simulink model "OUR_BD_FUELCELL"  (R2022b)
settings: Solver=ode1  StartTime=0.0  StopTime=max(cyc_mph(:,1))  FixedStep=1  MaxStep=1  RelTol=1e-3  AbsTol=1e-3
values from neighbouring files (symbols this model uses):
  eta_DC_DC = 1    [main.m]
  fc_pwr_scale = 0.6    [fuelcell_patch.m]
  Ts = 1    [main.m]
undefined symbols (not defined in the file or in its folder): air_cp, amb_tmp, cs_charge_deplete_bool, cs_charge_pwr, cs_fc_init_state, cs_fc_on, cs_hi_soc, cs_lo_soc, cs_max_pwr, cs_max_pwr_fall_rate, cs_max_pwr_rise_rate, cs_min_off_time, cs_min_pwr, ess_on, ex_calc, ex_gas_cp, fc_acc_mass, fc_base_mass, fc_c2i_th_cond, fc_c_init_tmp, fc_cl2h_eff, fc_co_map, fc_co_map_c2h, fc_cold, fc_cold_tmp, fc_cp, fc_eff_scale, fc_emis, fc_emisv, fc_exflow_map, fc_ext_sarea, fc_extmp_map, fc_fuel_den, fc_fuel_lhv, fc_fuel_map, fc_fuel_map_c2h, fc_fuelcell_warmup_bool, fc_h2x_th_cond, fc_h_air_flow, fc_h_cp, fc_h_init_tmp, fc_hc_map, fc_hc_map_c2h, fc_hood_emisv, fc_hood_sarea, fc_i2x_th_cond, fc_i_init_tmp, fc_nox_map, fc_nox_map_c2h, fc_o2_map, fc_on, fc_pm_map, fc_pm_map_c2h, fc_pwr_map, fc_tstat, fc_x_init_tmp, pow, veh_glider_mass
libraries: lib_wheel x2, lib_help x2, lib_transmission x2, lib_outputs x1, lib_controls x1, lib_interactive x1, lib_drive_cycle x1, lib_accessory x1, lib_energy_storage x1, lib_exhaust x1, mpclib x1, lib_electric_machine x1
(part 2 of 2)

== system OUR_BD_FUELCELL/fuel converter <fc> net model/fuel use and EO emis Fuel Cell/fc temp correct ==
  Coolant T (C) : Inport
  HOT fuel use (g/s) : Inport  Port=2
  HOT emis (g/s) : Inport  Port=3
  P (W) : Inport  Port=4
  Enable : EnablePort  StatesWhenEnabling=reset
  =1: use map based =0: use constant equation based : Constant  Value=fc_cold
  Switch : Switch  Threshold=eps
  Switch1 : Switch  Threshold=eps
  fc temp correct Constant Correction Factors (Equation Based) : Subsystem  TreatAsAtomicUnit=on
  fc temp correct Variable Correction Factors (Map Based) : Subsystem  TreatAsAtomicUnit=on
  fc_cold=0 : Logic  Operator=NOT
  fuel use (g/s) : Outport  OutputWhenDisabled=reset  InitialOutput=0
  EO emis (g/s) : Outport  Port=2  OutputWhenDisabled=reset  InitialOutput=0
  wires:
  Switch1/1 -> EO emis (g/s)/1
  Switch/1 -> fuel use (g/s)/1
  fc temp correct Variable Correction Factors (Map Based)/2(EO emis (g/s)) -> Switch1/3
  fc temp correct Constant Correction Factors (Equation Based)/2(EO emis (g/s)) -> Switch1/1
  fc temp correct Variable Correction Factors (Map Based)/1(fuel use (g/s)) -> Switch/3
  fc_cold=0/1 -> Switch1/2, Switch/2, fc temp correct Constant Correction Factors (Equation Based)/Enable
  fc temp correct Constant Correction Factors (Equation Based)/1(fuel use (g/s)) -> Switch/1
  HOT emis (g/s)/1 -> fc temp correct Variable Correction Factors (Map Based)/3(HOT emis (g/s)), fc temp correct Constant Correction Factors (Equation Based)/3(HOT emis (g/s))
  HOT fuel use (g/s)/1 -> fc temp correct Variable Correction Factors (Map Based)/2(HOT fuel use (g/s)), fc temp correct Constant Correction Factors (Equation Based)/2(HOT fuel use (g/s))
  Coolant T (C)/1 -> fc temp correct Variable Correction Factors (Map Based)/1(Coolant T (C)), fc temp correct Constant Correction Factors (Equation Based)/1(Coolant T (C))
  =1: use map based =0: use constant equation based/1 -> fc temp correct Variable Correction Factors (Map Based)/Enable, fc_cold=0/1
  P (W)/1 -> fc temp correct Variable Correction Factors (Map Based)/4(P (W))

== system OUR_BD_FUELCELL/fuel cell control strategy <cs>/FC on/no-lag Reset Integrator/dt ==
  Clock : Clock
  Memory1 : Memory  InitialCondition=-1
  Sum1 : Sum  Inputs=+-  InputSameDT=on  SaturateOnIntegerOverflow=on  OutDataTypeStr=Inherit: Same as first input
  out_1 : Outport  InitialOutput=0
  wires:
  Sum1/1 -> out_1/1
  Memory1/1 -> Sum1/2
  Clock/1 -> Memory1/1, Sum1/1

== system OUR_BD_FUELCELL/fuel cell control strategy <cs>/FC on1/no-lag Reset Integrator/dt ==
  Clock : Clock
  Memory1 : Memory  InitialCondition=-1
  Sum1 : Sum  Inputs=+-  InputSameDT=on  SaturateOnIntegerOverflow=on  OutDataTypeStr=Inherit: Same as first input
  out_1 : Outport  InitialOutput=0
  wires:
  Sum1/1 -> out_1/1
  Memory1/1 -> Sum1/2
  Clock/1 -> Memory1/1, Sum1/1

== system OUR_BD_FUELCELL/fuel converter <fc> net model/fuel cell system <fc>/pwr vs. eff fuel cell model/enforce limits ==
  In1 : Inport
  Gain : Gain  Gain=eta_DC_DC
  Saturation : Saturate  UpperLimit=max(fc_pwr_map)*fc_pwr_scale  LowerLimit=0
  Out1 : Outport  InitialOutput=0
  wires:
  In1/1 -> Saturation/1
  Saturation/1 -> Gain/1
  Gain/1 -> Out1/1

== system OUR_BD_FUELCELL/fuel converter <fc> net model/fuel use and EO emis Fuel Cell/HOT engine maps /Block NOTES ==
  note: This block determines the fully hot fuel use, engine-out emissions output rates, exhaust gas mass flow rate,
      | and engine-out exhaust gas temperature as a function of engine output torque and speed.
      | The engine maps (except for exhaust gas temperature) can be scaled using variables fc_spd_scale and
      |  fc_trq_scale; it is recommended that scaling values outside the range of 0.85 to 1.15 be used CAREFULLY.

== system OUR_BD_FUELCELL/fuel converter <fc> net model/fuel use and EO emis Fuel Cell/fc temp/Block NOTES ==
  note: This block models the thermal behavior internal combustion engine (ICE).
      | Emphasis is on the coolant since this temperature is used to correct engine
      | fuel use.

== system OUR_BD_FUELCELL/fuel converter <fc> net model/fuel use and EO emis Fuel Cell/fc temp/fc coolant ==
  Tcl : Inport
  "Qfc_i " : Inport  Port=2
  Enable : EnablePort  StatesWhenEnabling=reset
  Constant : Constant  Value=fc_tstat
  Product1 : Product  InputSameDT=on  RndMeth=Zero  SaturateOnIntegerOverflow=on  OutDataTypeStr=Inherit: Same as first input
  Qhtr : Fcn  Expr=fc_cl2h_eff*fc_h_air_flow*air_cp*(u - amb_tmp)
  Qi : Sum  Inputs=-+  InputSameDT=on  SaturateOnIntegerOverflow=on  OutDataTypeStr=Inherit: Same as first input
  Relational Operator : RelationalOperator  Operator=<=
  Qfc_rad : Outport  OutputWhenDisabled=reset  InitialOutput=0
  Qfc_htr : Outport  Port=2  OutputWhenDisabled=reset  InitialOutput=0
  wires:
  Qi/1 -> Product1/2
  Qhtr/1 -> Qfc_htr/1, Qi/1
  "Qfc_i "/1 -> Qi/2
  Product1/1 -> Qfc_rad/1
  Constant/1 -> Relational Operator/1
  Relational Operator/1 -> Product1/1
  Tcl/1 -> Relational Operator/2, Qhtr/1

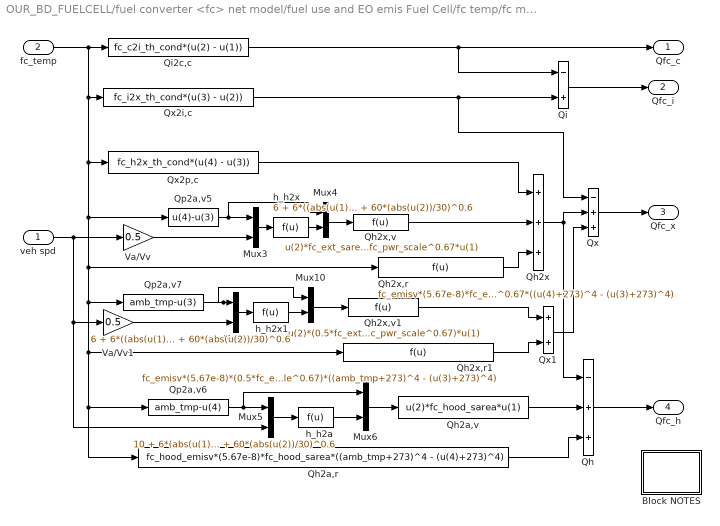
== system OUR_BD_FUELCELL/fuel converter <fc> net model/fuel use and EO emis Fuel Cell/fc temp/fc mass heat flow ==
  veh spd : Inport
  fc_temp : Inport  Port=2
  Block NOTES : Subsystem
      mask Display: disp('Block\nNOTES')
  Mux{3..6,9..10} (6 alike) : Mux  Inputs=2
  Qh : Sum  Inputs=-++  InputSameDT=on  SaturateOnIntegerOverflow=on  OutDataTypeStr=Inherit: Same as first input
  Qh2a,r : Fcn  Expr=fc_hood_emisv*(5.67e-8)*fc_hood_sarea*((amb_tmp+273)^4 - (u(4)+273)^4)
  Qh2a,v : Fcn  Expr=u(2)*fc_hood_sarea*u(1)
  Qh2x : Sum  Inputs=+++  InputSameDT=on  SaturateOnIntegerOverflow=on  OutDataTypeStr=Inherit: Same as first input
  Qh2x,r : Fcn  Expr=fc_emisv*(5.67e-8)*fc_ext_sarea*fc_pwr_scale^0.67*((u(4)+273)^4 - (u(3)+273)^4)
  Qh2x,r1 : Fcn  Expr=fc_emisv*(5.67e-8)*(0.5*fc_ext_sarea*fc_pwr_scale^0.67)*((amb_tmp+273)^4 - (u(3)+273)^4)
  Qh2x,v : Fcn  Expr=u(2)*fc_ext_sarea*fc_pwr_scale^0.67*u(1)
  Qh2x,v1 : Fcn  Expr=u(2)*(0.5*fc_ext_sarea*fc_pwr_scale^0.67)*u(1)
  Qi : Sum  Inputs=-+  InputSameDT=on  SaturateOnIntegerOverflow=on  OutDataTypeStr=Inherit: Same as first input
  Qi2c,c : Fcn  Expr=fc_c2i_th_cond*(u(2) - u(1))
  Qp2a,v5 : Fcn  Expr=u(4)-u(3)
  Qp2a,v6 : Fcn  Expr=amb_tmp-u(4)
  Qp2a,v7 : Fcn  Expr=amb_tmp-u(3)
  Qx : Sum  Inputs=-++  InputSameDT=on  SaturateOnIntegerOverflow=on  OutDataTypeStr=Inherit: Same as first input
  Qx1 : Sum  InputSameDT=on  SaturateOnIntegerOverflow=on  OutDataTypeStr=Inherit: Same as first input
  Qx2i,c : Fcn  Expr=fc_i2x_th_cond*(u(3) - u(2))
  Qx2p,c : Fcn  Expr=fc_h2x_th_cond*(u(4) - u(3))
  Va/Vv : Gain  Gain=0.5  SaturateOnIntegerOverflow=on  OutDataTypeStr=Inherit: Same as input  ParamDataTypeStr=Inherit: Same as input
  Va/Vv1 : Gain  Gain=0.5  SaturateOnIntegerOverflow=on  OutDataTypeStr=Inherit: Same as input  ParamDataTypeStr=Inherit: Same as input
  h_h2a : Fcn  Expr=10 + 6*(abs(u(1))/1000)^0.3 + 60*(abs(u(2))/30)^0.6
  h_h2x : Fcn  Expr=6 + 6*((abs(u(1))/1000))^0.3 + 60*(abs(u(2))/30)^0.6
  h_h2x1 : Fcn  Expr=6 + 6*((abs(u(1))/1000))^0.3 + 60*(abs(u(2))/30)^0.6
  Qfc_c : Outport
  Qfc_i : Outport  Port=2
  Qfc_x : Outport  Port=3
  Qfc_h : Outport  Port=4
  wires:
  Qh2x,r/1 -> Qh2x/3
  Qh2a,v/1 -> Qh/2
  Qh2a,r/1 -> Qh/3
  Qh2x,v1/1 -> Qx1/1
  Qh2x,r1/1 -> Qx1/2
  Qx2p,c/1 -> Qh2x/1
  Qh2x,v/1 -> Qh2x/2
  Qx1/1 -> Qx/3
  h_h2a/1 -> Mux6/2
  Qp2a,v6/1 -> Mux6/1, Mux5/1
  Mux5/1 -> h_h2a/1
  Mux6/1 -> Qh2a,v/1
  Qh/1 -> Qfc_h/1
  Qh2x/1 -> Qh/1, Qx/2
  Qx/1 -> Qfc_x/1
  Qi/1 -> Qfc_i/1
  Qx2i,c/1 -> Qx/1, Qi/2
  fc_temp/1 -> Qi2c,c/1, Qx2i,c/1, Qp2a,v5/1, Qh2x,r1/1, Qh2a,r/1, Qp2a,v6/1, Qp2a,v7/1, Qh2x,r/1, Qx2p,c/1
  Qi2c,c/1 -> Qi/1, Qfc_c/1
  Va/Vv/1 -> Mux3/2
  veh spd/1 -> Va/Vv1/1, Mux5/2, Va/Vv/1
  h_h2x/1 -> Mux4/2
  Qp2a,v5/1 -> Mux4/1, Mux3/1
  Mux3/1 -> h_h2x/1
  Mux4/1 -> Qh2x,v/1
  Va/Vv1/1 -> Mux9/2
  h_h2x1/1 -> Mux10/2
  Qp2a,v7/1 -> Mux10/1, Mux9/1
  Mux9/1 -> h_h2x1/1
  Mux10/1 -> Qh2x,v1/1

== system OUR_BD_FUELCELL/fuel converter <fc> net model/fuel use and EO emis Fuel Cell/fc temp/old fc coolant temp. (C) ==
  fc on? : Inport
  veh spd : Inport  Port=2
  Block NOTES : Subsystem
      mask Display: disp('Block\nNOTES')
  Mux : Mux
  TEC : Integrator  InitialCondition=fc_i_init_tmp
  compute engine dT/dt : Fcn  Expr=1.1*u[1]*(-u[2]/218)*(95-u[4])+(1-u[1])*u[3]*(u[4]-amb_tmp)
  gamma (takes v as input) : Fcn  Expr=(-8.22e-5*u+8.09e-6*4-1.45e-4)*.45
  log(1-40/75) : Constant  Value=-0.7621
  fc coolant temp (C) : Outport  InitialOutput=0
  wires:
  TEC/1 -> Mux/4, fc coolant temp (C)/1
  veh spd/1 -> gamma (takes v as input)/1
  fc on?/1 -> Mux/1
  Mux/1 -> compute engine dT/dt/1
  log(1-40/75)/1 -> Mux/2
  gamma (takes v as input)/1 -> Mux/3
  compute engine dT/dt/1 -> TEC/1

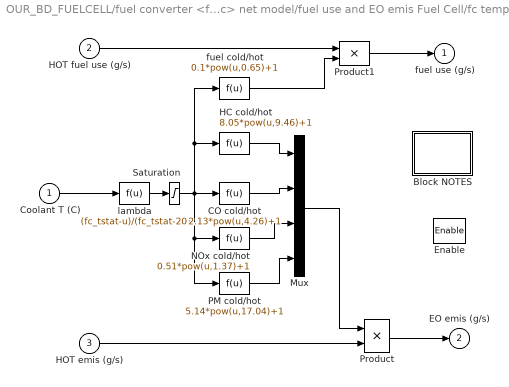
== system OUR_BD_FUELCELL/fuel converter <fc> net model/fuel use and EO emis Fuel Cell/fc temp correct/fc temp correct Constant Correction Factors (Equation Based) ==
  Coolant T (C) : Inport
  HOT fuel use (g/s) : Inport  Port=2
  HOT emis (g/s) : Inport  Port=3
  Enable : EnablePort  StatesWhenEnabling=reset
  Block NOTES : Subsystem
      mask Display: disp('Block\nNOTES')
  CO cold/hot : Fcn  Expr=2.13*pow(u,4.26)+1
  HC cold/hot : Fcn  Expr=8.05*pow(u,9.46)+1
  Mux : Mux
  NOx cold/hot : Fcn  Expr=0.51*pow(u,1.37)+1
  PM cold/hot : Fcn  Expr=5.14*pow(u,17.04)+1
  Product : Product  InputSameDT=on  RndMeth=Zero  SaturateOnIntegerOverflow=on  OutDataTypeStr=Inherit: Same as first input
  Product1 : Product  InputSameDT=on  RndMeth=Zero  SaturateOnIntegerOverflow=on  OutDataTypeStr=Inherit: Same as first input
  Saturation : Saturate  UpperLimit=1  LowerLimit=0
  fuel cold/hot : Fcn  Expr=0.1*pow(u,0.65)+1
  lambda : Fcn  Expr=(fc_tstat-u)/(fc_tstat-20)
  fuel use (g/s) : Outport  OutputWhenDisabled=reset  InitialOutput=0
  EO emis (g/s) : Outport  Port=2  OutputWhenDisabled=reset  InitialOutput=0
  wires:
  PM cold/hot/1 -> Mux/4
  NOx cold/hot/1 -> Mux/3
  HC cold/hot/1 -> Mux/1
  Saturation/1 -> CO cold/hot/1, HC cold/hot/1, fuel cold/hot/1, NOx cold/hot/1, PM cold/hot/1
  lambda/1 -> Saturation/1
  Mux/1 -> Product/1
  fuel cold/hot/1 -> Product1/2
  Product/1 -> EO emis (g/s)/1
  CO cold/hot/1 -> Mux/2
  Product1/1 -> fuel use (g/s)/1
  HOT fuel use (g/s)/1 -> Product1/1
  Coolant T (C)/1 -> lambda/1
  HOT emis (g/s)/1 -> Product/2

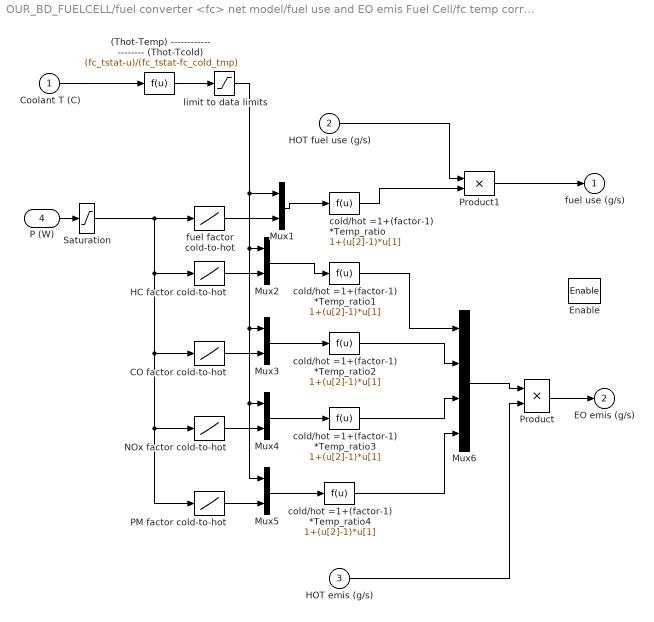
== system OUR_BD_FUELCELL/fuel converter <fc> net model/fuel use and EO emis Fuel Cell/fc temp correct/fc temp correct Variable Correction Factors (Map Based) ==
  Coolant T (C) : Inport
  HOT fuel use (g/s) : Inport  Port=2
  HOT emis (g/s) : Inport  Port=3
  P (W) : Inport  Port=4
  Enable : EnablePort  StatesWhenEnabling=reset
  (Thot-Temp) -------------------- (Thot-Tcold) : Fcn  Expr=(fc_tstat-u)/(fc_tstat-fc_cold_tmp)
  CO factor cold-to-hot : Lookup  InputValues=fc_pwr_map*fc_pwr_scale  Table=fc_co_map_c2h
  HC factor cold-to-hot : Lookup  InputValues=fc_pwr_map*fc_pwr_scale  Table=fc_hc_map_c2h
  Mux{1..5} (5 alike) : Mux  Inputs=2
  Mux6 : Mux
  NOx factor cold-to-hot : Lookup  InputValues=fc_pwr_map*fc_pwr_scale  Table=fc_nox_map_c2h
  PM factor cold-to-hot : Lookup  InputValues=fc_pwr_map*fc_pwr_scale  Table=fc_pm_map_c2h
  Product : Product  InputSameDT=on  RndMeth=Zero  SaturateOnIntegerOverflow=on  OutDataTypeStr=Inherit: Same as first input
  Product1 : Product  InputSameDT=on  RndMeth=Zero  SaturateOnIntegerOverflow=on  OutDataTypeStr=Inherit: Same as first input
  Saturation : Saturate  UpperLimit=max(fc_pwr_map*fc_pwr_scale)  LowerLimit=0
  cold/hot =1+(factor-1) *Temp_ratio{,1..4} (5 alike) : Fcn  Expr=1+(u[2]-1)*u[1]
  fuel factor cold-to-hot : Lookup  InputValues=fc_pwr_map*fc_pwr_scale  Table=fc_fuel_map_c2h
  limit to data limits : Saturate  UpperLimit=1  LowerLimit=0
  fuel use (g/s) : Outport  OutputWhenDisabled=reset  InitialOutput=0
  EO emis (g/s) : Outport  Port=2  OutputWhenDisabled=reset  InitialOutput=0
  wires:
  Mux6/1 -> Product/1
  HOT emis (g/s)/1 -> Product/2
  Product/1 -> EO emis (g/s)/1
  Product1/1 -> fuel use (g/s)/1
  Mux5/1 -> cold/hot =1+(factor-1) *Temp_ratio4/1
  Mux4/1 -> cold/hot =1+(factor-1) *Temp_ratio3/1
  Mux3/1 -> cold/hot =1+(factor-1) *Temp_ratio2/1
  Mux2/1 -> cold/hot =1+(factor-1) *Temp_ratio1/1
  PM factor cold-to-hot/1 -> Mux5/2
  NOx factor cold-to-hot/1 -> Mux4/2
  CO factor cold-to-hot/1 -> Mux3/2
  HC factor cold-to-hot/1 -> Mux2/2
  Mux1/1 -> cold/hot =1+(factor-1) *Temp_ratio/1
  fuel factor cold-to-hot/1 -> Mux1/2
  Coolant T (C)/1 -> (Thot-Temp) -------------------- (Thot-Tcold)/1
  HOT fuel use (g/s)/1 -> Product1/1
  P (W)/1 -> Saturation/1
  Saturation/1 -> fuel factor cold-to-hot/1, HC factor cold-to-hot/1, CO factor cold-to-hot/1, NOx factor cold-to-hot/1, PM factor cold-to-hot/1
  (Thot-Temp) -------------------- (Thot-Tcold)/1 -> limit to data limits/1
  limit to data limits/1 -> Mux5/1, Mux4/1, Mux3/1, Mux2/1, Mux1/1
  cold/hot =1+(factor-1) *Temp_ratio/1 -> Product1/2
  cold/hot =1+(factor-1) *Temp_ratio1/1 -> Mux6/1
  cold/hot =1+(factor-1) *Temp_ratio2/1 -> Mux6/2
  cold/hot =1+(factor-1) *Temp_ratio3/1 -> Mux6/3
  cold/hot =1+(factor-1) *Temp_ratio4/1 -> Mux6/4

== system OUR_BD_FUELCELL/fuel converter <fc> net model/fuel use and EO emis Fuel Cell/fc temp/fc mass heat flow/Block NOTES ==
  note: FUEL CONVERTER MASS HEAT LOSS
      | This block models the heat loss from a fuel converter (such as an IC engine).
      | Convection (as a function of vehicle speed), radiation, and conduction effects are included.
      | Engine cylinder (c), interior (i), exterior (x) and hood (h)
      | heat flows are estimated based on the temperatures from the previous iteration.

== system OUR_BD_FUELCELL/fuel converter <fc> net model/fuel use and EO emis Fuel Cell/fc temp/old fc coolant temp. (C)/Block NOTES ==
  note: This block computes engine coolant temperature,
      | assuming that it asymptotically approaches its maximum
      | temperature when the engine is on, and asymptotically
      | approaches the ambient temperature when the engine
      | is off.  Temperatue rise rate is assumed to be a function
      | only of current engine coolant temperature, and the fall
      | rate is also a function of vehicle speed and ambient temperature.
      | There is no dependence on engine load or speed.

== system OUR_BD_FUELCELL/fuel converter <fc> net model/fuel use and EO emis Fuel Cell/fc temp correct/fc temp correct Constant Correction Factors (Equation Based)/Block NOTES ==
  note: This block determines actual fuel use and engine-out emissions
      | given the fully hot values and the engine coolant temperature.
      | The correlations used here were developed at NREL using
      | Hot and Cold Engine data collected
      | at Oak Ridge National Laboratory.
